simulink model "test"  (Simulink 7.5)
settings: Solver=ode45  StartTime=0.0  StopTime=10.0  RelTol=1e-3
InitFcn:
  | %% DSPBuilder Start
  | alt_dspbuilder_update_model(bdroot)
  | %% DSPBuilder End
libraries: allblocks_alteradspbuilder2 x7
settings Model: Creator=Administrator  LastModifiedBy=Administrator

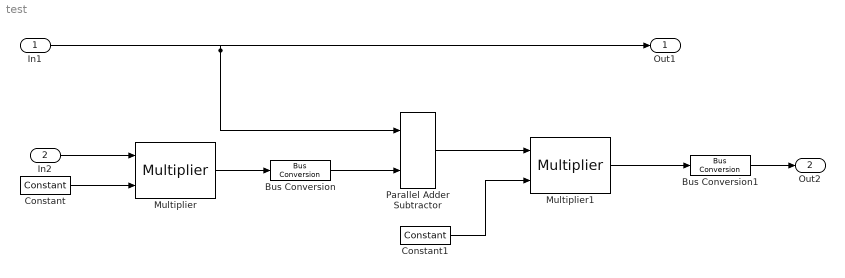
== system test ==
  In1 : Inport  OutDataType=fixdt(1, 16)  OutScaling=2^0
  In2 : Inport  Port=2  OutDataType=fixdt(1, 16)  OutScaling=2^0
  Bus Conversion : allblocks_alteradspbuilder2/Bus Conversion  BusType=Signed Fractional  ibwl=18  ibwr=14  bwl=2  bwr=14  bitToConnectToOutputLSB=3  round=off  saturate=off  pipeline_display=0
  Bus Conversion1 : allblocks_alteradspbuilder2/Bus Conversion  BusType=Signed Fractional  ibwl=4  ibwr=28  bwl=2  bwr=14  bitToConnectToOutputLSB=3  round=off  saturate=off  pipeline_display=0
  Constant : allblocks_alteradspbuilder2/Constant  mask_cst=2  BusType=Signed Integer  bwl=16  bwr=0  roundMode=Truncate  satMode=Wrap  SpecifyClock=off  allowFloatingPointOverride=on  logOutputs=off  logFile=C:\altera\13.1\quartus\dsp_builder\tb_test\test_Constant.fixedpointlog
  Constant1 : allblocks_alteradspbuilder2/Constant  mask_cst=sqrt(1/3)  BusType=Signed Fractional  bwl=2  bwr=14  roundMode=Truncate  satMode=Wrap  SpecifyClock=off  allowFloatingPointOverride=on  logOutputs=off  logFile=C:\altera\13.1\quartus\dsp_builder\tb_test\test_Constant1.fixedpointlog
  Multiplier : allblocks_alteradspbuilder2/Multiplier  BusType=Signed Fractional  bwl=2  bwr=14  pipeline=0  pipeline_display=0  allowFloatingPointOverride=on  logOutputs=off  logFile=C:\altera\13.1\quartus\dsp_builder\tb_test\test_Multiplier.fixedpointlog  UseEqualInputWidth=off  bbwl=16  bbwr=0  FullResolution=on  OutputMsb=8  OutputLsb=0  OutputBwl=16  OutputBwr=16  UseDedicatedCircuitry=YES  use_ena=off  use_aclr=off
  Multiplier1 : allblocks_alteradspbuilder2/Multiplier  BusType=Signed Fractional  bwl=2  bwr=14  pipeline=0  pipeline_display=0  allowFloatingPointOverride=on  logOutputs=off  logFile=C:\altera\13.1\quartus\dsp_builder\tb_test\test_Multiplier1.fixedpointlog  UseEqualInputWidth=off  bbwl=2  bbwr=14  FullResolution=on  OutputMsb=8  OutputLsb=0  OutputBwl=16  OutputBwr=16  UseDedicatedCircuitry=YES  use_ena=off  use_aclr=off
  Parallel Adder Subtractor : allblocks_alteradspbuilder2/Parallel Adder Subtractor  number_of_inputs=2  direction=++  use_pipeline=on  pipeline_display=1  phase_selection=1  use_ena=off  use_aclr=off  allowFloatingPointOverride=on  logOutputs=off  logFile=C:\altera\13.1\quartus\dsp_builder\tb_test\test_Parallel+Adder+Subtractor.fixedpointlog
  Out1 : Outport  OutDataType=fixdt(1, 16)  OutScaling=2^0
  Out2 : Outport  Port=2  OutDataType=fixdt(1, 16)  OutScaling=2^0
  wires:
  In2/1 -> Multiplier/1
  Constant/1 -> Multiplier/2
  Multiplier/1 -> Bus Conversion/1
  Bus Conversion/1 -> Parallel Adder Subtractor/2
  In1/1 -> Parallel Adder Subtractor/1, Out1/1
  Constant1/1 -> Multiplier1/2
  Parallel Adder Subtractor/1 -> Multiplier1/1
  Multiplier1/1 -> Bus Conversion1/1
  Bus Conversion1/1 -> Out2/1
